simulink model "ThdRwStOccupyChk"  (R2018b)
settings: Solver=FixedStepDiscrete  StartTime=0.0  StopTime=10.0  FixedStep=0.01  RelTol=1e-3
undefined symbols (not defined in the file or in its folder): SeatOccupiedSts1
settings Model: Creator=sn2xws  LastModifiedBy=sn2xws
settings Model: ModifiedHistory=|
  | 2024.9.11 V3.0.0
  | BUG 910711 三左三中任意1个占座，则判断为三左占座
settings DataIOCC: SaveFormat=StructureWithTime
settings OptimizationCC: DefaultParameterBehavior=Inlined  EnhancedBackFolding=on  PassReuseOutputArgsAs=Individual arguments  ZeroExternalMemoryAtStartup=off  ZeroInternalMemoryAtStartup=off  OptimizeBlockOrder=speed  DifferentSizesBufferReuse=on  OptimizationCustomize=off
settings DebuggingCC: ParameterTunabilityLossMsg=error
settings ModelReferenceCC: ModelReferenceNumInstancesAllowed=Single
settings SFSimCC: MATLABDynamicMemAlloc=off
settings RTWCC: SystemTargetFile=autosar.tlc  GenCodeOnly=on  TemplateMakefile=ert_default_tmf  Description=AUTOSAR  GenerateReport=on  IncludeHyperlinkInReport=on  LaunchReport=on  GenerateTraceInfo=on  GenerateTraceReport=on  GenerateTraceReportSl=on  GenerateTraceReportSf=on  GenerateTraceReportEml=on
settings CodeAppCC: ForceParamTrailComments=on  IgnoreCustomStorageClasses=off  OperatorAnnotations=on  SimulinkDataObjDesc=on  SFDataObjDesc=on  InsertBlockDesc=on
settings STFCustomTargetCC: TargetLangStandard=C99 (ISO)  MultiwordLength=256  ParMdlRefBuildCompliant=on  CompOptLevelCompliant=on  IncludeMdlTerminateFcn=off  CombineOutputUpdateFcns=on  SuppressErrorStatus=on  ERTCustomFileBanners=on  SupportNonFinite=off  SupportComplex=off  SupportContinuousTime=off  SupportNonInlinedSFcns=off  RemoveResetFunc=on  MATLABClassNameForMDSCustomization=Simulink.SoftwareTarget.ERTCustomization  AutosarCompliant=on  UseToolchainInfoCompliant=on  LookupTableObjectStructAxisOrder=2,1,3,4,...  LUTObjectStructOrderEvenSpacing=Size,Table,Breakpoints  SystemTargetFile=autosar.tlc
settings ERTTargetCC: TargetLangStandard=C99 (ISO)  ConcurrentExecutionCompliant=off  IncludeMdlTerminateFcn=off  SuppressErrorStatus=on  SupportNonFinite=off  SupportComplex=off  ModelStepFunctionPrototypeControlCompliant=off  CPPClassGenCompliant=off  AutosarCompliant=on  LookupTableObjectStructAxisOrder=2,1,3,4,...  LUTObjectStructOrderEvenSpacing=Size,Table,Breakpoints  InlinedParameterPlacement=NonHierarchical  ERTCustomFileTemplate=example_file_process.tlc  ERTFilePackagingFormat=Compact

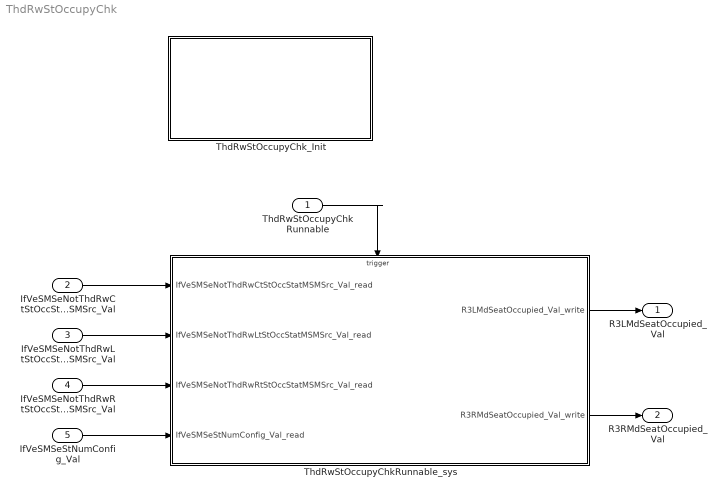
== system ThdRwStOccupyChk ==
  ThdRwStOccupyChkRunnable : Inport  SampleTime=0.01  OutputFunctionCall=on
  IfVeSMSeNotThdRwCtStOccStatMSMSrc_Val : Inport  Port=2  OutDataTypeStr=Enum: SeatOccupiedSts1  PortDimensions=1
  IfVeSMSeNotThdRwLtStOccStatMSMSrc_Val : Inport  Port=3  OutDataTypeStr=Enum: SeatOccupiedSts1  PortDimensions=1
  IfVeSMSeNotThdRwRtStOccStatMSMSrc_Val : Inport  Port=4  OutDataTypeStr=Enum: SeatOccupiedSts1  PortDimensions=1
  IfVeSMSeStNumConfig_Val : Inport  Port=5  OutDataTypeStr=Enum: IfVeSMSeStNumConfig  PortDimensions=1
  ThdRwStOccupyChkRunnable_sys : Subsystem
  ThdRwStOccupyChk_Init : Subsystem
  R3LMdSeatOccupied_Val : Outport  OutDataTypeStr=boolean  PortDimensions=1
  R3RMdSeatOccupied_Val : Outport  Port=2  OutDataTypeStr=boolean  PortDimensions=1
  wires:
  IfVeSMSeNotThdRwCtStOccStatMSMSrc_Val/1 -> ThdRwStOccupyChkRunnable_sys/1(IfVeSMSeNotThdRwCtStOccStatMSMSrc_Val_read)
  IfVeSMSeNotThdRwLtStOccStatMSMSrc_Val/1 -> ThdRwStOccupyChkRunnable_sys/2(IfVeSMSeNotThdRwLtStOccStatMSMSrc_Val_read)
  IfVeSMSeNotThdRwRtStOccStatMSMSrc_Val/1 -> ThdRwStOccupyChkRunnable_sys/3(IfVeSMSeNotThdRwRtStOccStatMSMSrc_Val_read)
  IfVeSMSeStNumConfig_Val/1 -> ThdRwStOccupyChkRunnable_sys/4(IfVeSMSeStNumConfig_Val_read)
  ThdRwStOccupyChkRunnable_sys/1(R3LMdSeatOccupied_Val_write) -> R3LMdSeatOccupied_Val/1
  ThdRwStOccupyChkRunnable_sys/2(R3RMdSeatOccupied_Val_write) -> R3RMdSeatOccupied_Val/1
  ThdRwStOccupyChkRunnable/1 -> ThdRwStOccupyChkRunnable_sys/Trigger

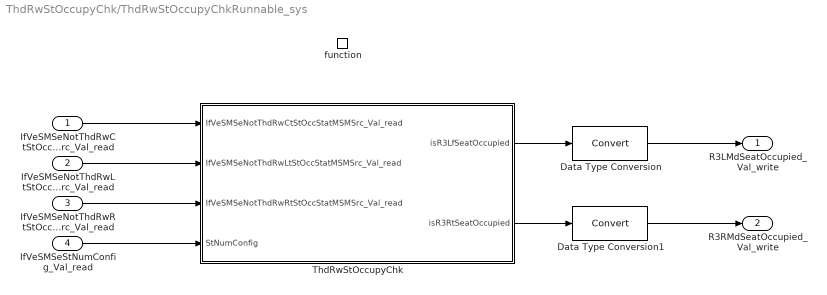
== system ThdRwStOccupyChk/ThdRwStOccupyChkRunnable_sys ==
  IfVeSMSeNotThdRwCtStOccStatMSMSrc_Val_read : Inport
  IfVeSMSeNotThdRwLtStOccStatMSMSrc_Val_read : Inport  Port=2
  IfVeSMSeNotThdRwRtStOccStatMSMSrc_Val_read : Inport  Port=3
  IfVeSMSeStNumConfig_Val_read : Inport  Port=4
  function : TriggerPort  TriggerType=function-call  VariantControl=(inherit)  SampleTimeType=periodic  SampleTime=-1
  Data Type Conversion : DataTypeConversion
  Data Type Conversion1 : DataTypeConversion
  ThdRwStOccupyChk : Subsystem
  R3LMdSeatOccupied_Val_write : Outport
      settings: EnsureOutportIsVirtual=on
  R3RMdSeatOccupied_Val_write : Outport  Port=2
      settings: EnsureOutportIsVirtual=on
  wires:
  IfVeSMSeNotThdRwCtStOccStatMSMSrc_Val_read/1 -> ThdRwStOccupyChk/1(IfVeSMSeNotThdRwCtStOccStatMSMSrc_Val_read)
  IfVeSMSeNotThdRwLtStOccStatMSMSrc_Val_read/1 -> ThdRwStOccupyChk/2(IfVeSMSeNotThdRwLtStOccStatMSMSrc_Val_read)
  IfVeSMSeNotThdRwRtStOccStatMSMSrc_Val_read/1 -> ThdRwStOccupyChk/3(IfVeSMSeNotThdRwRtStOccStatMSMSrc_Val_read)
  IfVeSMSeStNumConfig_Val_read/1 -> ThdRwStOccupyChk/4(StNumConfig)
  ThdRwStOccupyChk/1(isR3LfSeatOccupied) -> Data Type Conversion/1
  ThdRwStOccupyChk/2(isR3RtSeatOccupied) -> Data Type Conversion1/1
  Data Type Conversion/1 -> R3LMdSeatOccupied_Val_write/1
  Data Type Conversion1/1 -> R3RMdSeatOccupied_Val_write/1

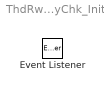
== system ThdRwStOccupyChk/ThdRwStOccupyChk_Init ==
  Event Listener : EventListener  EventName=reset

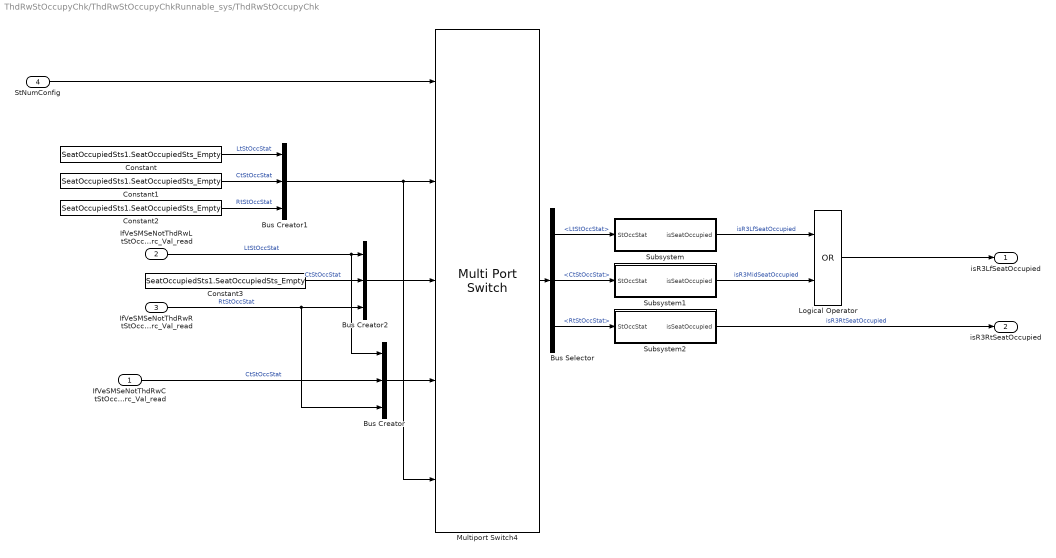
== system ThdRwStOccupyChk/ThdRwStOccupyChkRunnable_sys/ThdRwStOccupyChk ==
  IfVeSMSeNotThdRwCtStOccStatMSMSrc_Val_read : Inport
  IfVeSMSeNotThdRwLtStOccStatMSMSrc_Val_read : Inport  Port=2
  IfVeSMSeNotThdRwRtStOccStatMSMSrc_Val_read : Inport  Port=3
  StNumConfig : Inport  Port=4
  Bus Creator : BusCreator  Inputs=3
  Bus Creator1 : BusCreator  Inputs=3
  Bus Creator2 : BusCreator  Inputs=3
  Bus Selector : BusSelector  OutputSignals=LtStOccStat,CtStOccStat,RtStOccStat
  Constant{,1..3} (4 alike) : Constant  Value=SeatOccupiedSts1.SeatOccupiedSts_Empty  OutDataTypeStr=Enum:SeatOccupiedSts1
  Logical Operator : Logic  Operator=OR  AllPortsSameDT=off  OutDataTypeStr=boolean
  Multiport Switch4 : MultiPortSwitch  DataPortOrder=Specify indices  DataPortIndices={IfVeSMSeStNumConfig.SeatNum4Config,IfVeSMSeStNumConfig.SeatNum6Config,IfVeSMSeStNumConfig.SeatNum7Config,IfVeSMSeStNumConfig.SeatNum4PConfig}  DiagnosticForDefault=None
  Subsystem : Subsystem
  Subsystem1 : Subsystem
  Subsystem2 : Subsystem
  isR3LfSeatOccupied : Outport
  isR3RtSeatOccupied : Outport  Port=2
  wires:
  Subsystem/1(isSeatOccupied) -> Logical Operator/1  "isR3LfSeatOccupied"
  Subsystem2/1(isSeatOccupied) -> isR3RtSeatOccupied/1  "isR3RtSeatOccupied"
  StNumConfig/1 -> Multiport Switch4/1
  IfVeSMSeNotThdRwCtStOccStatMSMSrc_Val_read/1 -> Bus Creator/2  "CtStOccStat"
  Bus Creator/1 -> Multiport Switch4/4
  Multiport Switch4/1 -> Bus Selector/1
  Constant2/1 -> Bus Creator1/3  "RtStOccStat"
  Constant/1 -> Bus Creator1/1  "LtStOccStat"
  Bus Creator1/1 -> Multiport Switch4/2, Multiport Switch4/5
  Constant1/1 -> Bus Creator1/2  "CtStOccStat"
  Constant3/1 -> Bus Creator2/2  "CtStOccStat"
  Bus Creator2/1 -> Multiport Switch4/3
  IfVeSMSeNotThdRwLtStOccStatMSMSrc_Val_read/1 -> Bus Creator/1, Bus Creator2/1  "LtStOccStat"
  IfVeSMSeNotThdRwRtStOccStatMSMSrc_Val_read/1 -> Bus Creator2/3, Bus Creator/3  "RtStOccStat"
  Bus Selector/1 -> Subsystem/1(StOccStat)  "<LtStOccStat>"
  Bus Selector/2 -> Subsystem1/1(StOccStat)  "<CtStOccStat>"
  Bus Selector/3 -> Subsystem2/1(StOccStat)  "<RtStOccStat>"
  Subsystem1/1(isSeatOccupied) -> Logical Operator/2  "isR3MidSeatOccupied"
  Logical Operator/1 -> isR3LfSeatOccupied/1

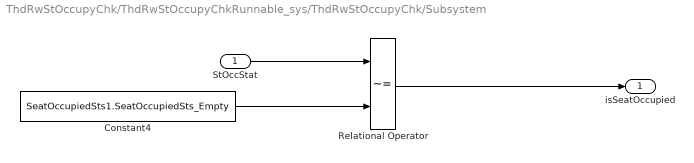
== system ThdRwStOccupyChk/ThdRwStOccupyChkRunnable_sys/ThdRwStOccupyChk/Subsystem ==
  StOccStat : Inport
  Constant4 : Constant  Value=SeatOccupiedSts1.SeatOccupiedSts_Empty  OutDataTypeStr=Enum:SeatOccupiedSts1
  Relational Operator : RelationalOperator  Operator=~=  OutDataTypeStr=boolean  RndMeth=Simplest
  isSeatOccupied : Outport  VectorParamsAs1DForOutWhenUnconnected=on
  wires:
  Constant4/1 -> Relational Operator/2
  StOccStat/1 -> Relational Operator/1
  Relational Operator/1 -> isSeatOccupied/1

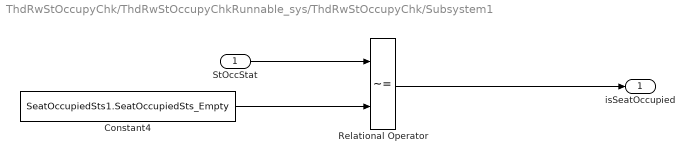
== system ThdRwStOccupyChk/ThdRwStOccupyChkRunnable_sys/ThdRwStOccupyChk/Subsystem1 ==
  StOccStat : Inport
  Constant4 : Constant  Value=SeatOccupiedSts1.SeatOccupiedSts_Empty  OutDataTypeStr=Enum:SeatOccupiedSts1
  Relational Operator : RelationalOperator  Operator=~=  OutDataTypeStr=boolean  RndMeth=Simplest
  isSeatOccupied : Outport  VectorParamsAs1DForOutWhenUnconnected=on
  wires:
  Relational Operator/1 -> isSeatOccupied/1
  StOccStat/1 -> Relational Operator/1
  Constant4/1 -> Relational Operator/2

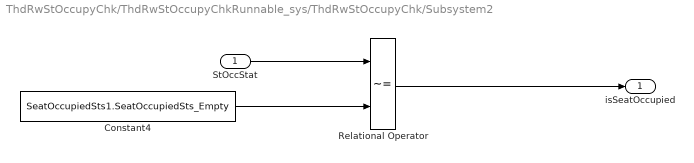
== system ThdRwStOccupyChk/ThdRwStOccupyChkRunnable_sys/ThdRwStOccupyChk/Subsystem2 ==
  StOccStat : Inport
  Constant4 : Constant  Value=SeatOccupiedSts1.SeatOccupiedSts_Empty  OutDataTypeStr=Enum:SeatOccupiedSts1
  Relational Operator : RelationalOperator  Operator=~=  OutDataTypeStr=boolean  RndMeth=Simplest
  isSeatOccupied : Outport  VectorParamsAs1DForOutWhenUnconnected=on
  wires:
  Constant4/1 -> Relational Operator/2
  StOccStat/1 -> Relational Operator/1
  Relational Operator/1 -> isSeatOccupied/1
